simulink model "torqueBalancing2015a"  (Simulink 8.5)
settings: Solver=FixedStepDiscrete  StartTime=0.0  StopTime="CONFIG.SIMULATION_TIME "  FixedStep=CONFIG.Ts  RelTol=1e-3
InitFcn:
  | cd(fileparts(which(bdroot)));
  | initTorqueBalancing;
values from neighbouring files (symbols this model uses):
  WBT_modelName = 'matlabTorqueBalancing'    [initTorqueBalancing.m]
undefined symbols (not defined in the file or in its folder): bVectorConstraintsFeet, bVectorConstraintsLegs, CONFIG, ConstraintsMatrixFeet, ConstraintsMatrixLegs, DiscIntNeverNeededParam, gain, references, reg, ROBOT_DOF, ROBOT_DOF_FOR_SIMULINK, sat, SM, sm, WBT_robotName
libraries: WBToolboxLibrary x177, simulink x13
(part 4 of 4)

== system torqueBalancing2015a/DesValues/State Machine StandUp/visualise inertial/l_sole_H_root_link3 ==
  qj : Inport
  Constant5 : Constant  Value=eye(4)
  Constant6 : Constant  Value=eye(4)
  Inv\* : Product  Inputs=/*  Multiplication=Matrix(*)
  Visualize hom transf4 : Subsystem
  link_name : WBToolboxLibrary/wholeBodyModel/Kinematics/Forward Kinematics  frameName=link_name  robotName=WBT_robotName  localName=WBT_modelName  wbiFile=WBT_wbiFilename  wbiList=WBT_wbiList
  root_link : WBToolboxLibrary/wholeBodyModel/Kinematics/Forward Kinematics  frameName='root_link'  robotName=WBT_robotName  localName=WBT_modelName  wbiFile=WBT_wbiFilename  wbiList=WBT_wbiList
  link_name_H_root_link : Outport
  wires:
  Constant5/1 -> link_name/1
  Inv\*/1 -> link_name_H_root_link/1  "link_name_H_root_link"
  link_name/1 -> Inv\*/1
  Constant6/1 -> root_link/1
  qj/1 -> link_name/2, root_link/2
  root_link/1 -> Visualize hom transf4/1(H), Inv\*/2

== system torqueBalancing2015a/DesValues/State Machine StandUp/visualise inertial/w_H_root_link1 ==
  qj : Inport
  inertial : Inport  Port=2
  "CoM6D ->  CoMXYZ1" : Selector  NumberOfDimensions=2  InputPortWidth=7  IndexOptions=Index vector (dialog),Index vector (dialog)  Indices=[1 2 3],[1 2 3]  OutputSizes=1,1
  Constant : Constant  Value=zeros(3,1)
  Constant2 : Constant  Value=eye(4)
  Constant5 : Constant  Value=eye(4)
  Constant6 : Constant  Value=eye(4)
  Gain : Gain  Gain=pi/180
  Head state : WBToolboxLibrary/Utilities/Yarp Read  portName=[WBT_robotName, '/head/state:o']  signalSize=6  blocking=off  timestamp=off  autoconnect=on  errorOnConnection=off
  Inv\* : Product  Inputs=/*  Multiplication=Matrix(*)
  Inv\*1 : Product  Inputs=/*  Multiplication=Matrix(*)
  Inv\*2 : Product  Inputs=/  Multiplication=Matrix(*)
  Product : Product  Multiplication=Matrix(*)
  Selector : Selector  InputPortWidth=12  IndexOptions=Index vector (dialog)  Indices=[4 5 6 ]  OutputSizes=1
  Selector1 : Selector  InputPortWidth=6  IndexOptions=Index vector (dialog)  Indices=[1:3]  OutputSizes=1
  Switch : Switch  Criteria=u2 > Threshold
  Switch6 : Switch  Criteria=u2 > Threshold
  USE_IMU4EST_BASE : Constant  Value=CONFIG.USE_IMU4EST_BASE
  USE_IMU4EST_BASE1 : Constant  Value=CONFIG.CORRECT_NECK_IMU
  fromImuToHomogeousTransformFCN : MATLAB Function  TreatAsAtomicUnit=on
      settings: PermitHierarchicalResolution=ParametersOnly
  holder 1 : WBToolboxLibrary/Utilities/holder 
  holder 2 : WBToolboxLibrary/Utilities/holder 
  imu : WBToolboxLibrary/wholeBodyModel/Kinematics/Forward Kinematics  frameName='imu_frame'  robotName=WBT_robotName  localName=WBT_modelName  wbiFile=WBT_wbiFilename  wbiList=WBT_wbiList
  l_sole_acc : Scope
      settings: TimeRange=60  ShowLegends=on  MaxDataPoints=5000  SaveToWorkspace=off  YMin=-4.47309  YMax=14.2668  SampleTime=-1
  link : WBToolboxLibrary/wholeBodyModel/Kinematics/Forward Kinematics  frameName=link_name  robotName=WBT_robotName  localName=WBT_modelName  wbiFile=WBT_wbiFilename  wbiList=WBT_wbiList
  root_link : WBToolboxLibrary/wholeBodyModel/Kinematics/Forward Kinematics  frameName='root_link'  robotName=WBT_robotName  localName=WBT_modelName  wbiFile=WBT_wbiFilename  wbiList=WBT_wbiList
  w_H_root : Outport
  wires:
  Constant5/1 -> imu/1
  Inv\*/1 -> Inv\*2/1, holder 1/1, fromImuToHomogeousTransformFCN/1(imu_H_link)  "imu_H_link"
  imu/1 -> Inv\*/1
  Constant6/1 -> link/1
  Inv\*1/1 -> Switch6/3, fromImuToHomogeousTransformFCN/3(link_H_root)  "link_H_root"
  link/1 -> Inv\*/2, Inv\*1/1
  inertial/1 -> Selector/1, holder 2/1, fromImuToHomogeousTransformFCN/5(inertial)
  Switch6/1 -> w_H_root/1
  USE_IMU4EST_BASE/1 -> Switch6/2
  fromImuToHomogeousTransformFCN/1(w_H_root) -> Switch6/1
  Constant2/1 -> root_link/1
  qj/1 -> root_link/2, link/2, imu/2
  root_link/1 -> Inv\*1/2
  holder 1/1 -> fromImuToHomogeousTransformFCN/2(imu_H_link_0)
  holder 2/1 -> fromImuToHomogeousTransformFCN/4(inertial_0)
  Inv\*2/1 -> "CoM6D ->  CoMXYZ1"/1
  "CoM6D ->  CoMXYZ1"/1 -> Product/1  "l_sole_R_imu"
  Selector/1 -> Product/2  "imu_acce"
  Product/1 -> l_sole_acc/1
  Head state/1 -> Gain/1
  Selector1/1 -> Switch/1  "neck"
  USE_IMU4EST_BASE1/1 -> Switch/2
  Switch/1 -> fromImuToHomogeousTransformFCN/6(neck)
  Gain/1 -> Selector1/1
  Constant/1 -> Switch/3

== system torqueBalancing2015a/DesValues/State Machine StandUp/visualise inertial/w_H_root_link4 ==
  qj : Inport
  inertial : Inport  Port=2
  "CoM6D ->  CoMXYZ1" : Selector  NumberOfDimensions=2  InputPortWidth=7  IndexOptions=Index vector (dialog),Index vector (dialog)  Indices=[1 2 3],[1 2 3]  OutputSizes=1,1
  Constant : Constant  Value=zeros(3,1)
  Constant2 : Constant  Value=eye(4)
  Constant5 : Constant  Value=eye(4)
  Constant6 : Constant  Value=eye(4)
  Gain : Gain  Gain=pi/180
  Head state : WBToolboxLibrary/Utilities/Yarp Read  portName=[WBT_robotName, '/head/state:o']  signalSize=6  blocking=off  timestamp=off  autoconnect=on  errorOnConnection=off
  Inv\* : Product  Inputs=/*  Multiplication=Matrix(*)
  Inv\*1 : Product  Inputs=/*  Multiplication=Matrix(*)
  Inv\*2 : Product  Inputs=/  Multiplication=Matrix(*)
  Product : Product  Multiplication=Matrix(*)
  Selector : Selector  InputPortWidth=12  IndexOptions=Index vector (dialog)  Indices=[4 5 6 ]  OutputSizes=1
  Selector1 : Selector  InputPortWidth=6  IndexOptions=Index vector (dialog)  Indices=[1:3]  OutputSizes=1
  Switch : Switch  Criteria=u2 > Threshold
  Switch6 : Switch  Criteria=u2 > Threshold
  USE_IMU4EST_BASE : Constant  Value=CONFIG.USE_IMU4EST_BASE
  USE_IMU4EST_BASE1 : Constant  Value=CONFIG.CORRECT_NECK_IMU
  fromImuToHomogeousTransformFCN : MATLAB Function  TreatAsAtomicUnit=on
      settings: PermitHierarchicalResolution=ParametersOnly
  holder 1 : WBToolboxLibrary/Utilities/holder 
  holder 2 : WBToolboxLibrary/Utilities/holder 
  imu : WBToolboxLibrary/wholeBodyModel/Kinematics/Forward Kinematics  frameName='imu_frame'  robotName=WBT_robotName  localName=WBT_modelName  wbiFile=WBT_wbiFilename  wbiList=WBT_wbiList
  l_sole_acc : Scope
      settings: TimeRange=60  ShowLegends=on  MaxDataPoints=5000  SaveToWorkspace=off  YMin=-4.47309  YMax=14.2668  SampleTime=-1
  link : WBToolboxLibrary/wholeBodyModel/Kinematics/Forward Kinematics  frameName=link_name  robotName=WBT_robotName  localName=WBT_modelName  wbiFile=WBT_wbiFilename  wbiList=WBT_wbiList
  root_link : WBToolboxLibrary/wholeBodyModel/Kinematics/Forward Kinematics  frameName='root_link'  robotName=WBT_robotName  localName=WBT_modelName  wbiFile=WBT_wbiFilename  wbiList=WBT_wbiList
  w_H_root : Outport
  wires:
  Constant5/1 -> imu/1
  Inv\*/1 -> Inv\*2/1, holder 1/1, fromImuToHomogeousTransformFCN/1(imu_H_link)  "imu_H_link"
  imu/1 -> Inv\*/1
  Constant6/1 -> link/1
  Inv\*1/1 -> Switch6/3, fromImuToHomogeousTransformFCN/3(link_H_root)  "link_H_root"
  link/1 -> Inv\*/2, Inv\*1/1
  inertial/1 -> Selector/1, holder 2/1, fromImuToHomogeousTransformFCN/5(inertial)
  Switch6/1 -> w_H_root/1
  USE_IMU4EST_BASE/1 -> Switch6/2
  fromImuToHomogeousTransformFCN/1(w_H_root) -> Switch6/1
  Constant2/1 -> root_link/1
  qj/1 -> root_link/2, link/2, imu/2
  root_link/1 -> Inv\*1/2
  holder 1/1 -> fromImuToHomogeousTransformFCN/2(imu_H_link_0)
  holder 2/1 -> fromImuToHomogeousTransformFCN/4(inertial_0)
  Inv\*2/1 -> "CoM6D ->  CoMXYZ1"/1
  "CoM6D ->  CoMXYZ1"/1 -> Product/1  "l_sole_R_imu"
  Selector/1 -> Product/2  "imu_acce"
  Product/1 -> l_sole_acc/1
  Head state/1 -> Gain/1
  Selector1/1 -> Switch/1  "neck"
  USE_IMU4EST_BASE1/1 -> Switch/2
  Switch/1 -> fromImuToHomogeousTransformFCN/6(neck)
  Gain/1 -> Selector1/1
  Constant/1 -> Switch/3

== system torqueBalancing2015a/DesValues/State Machine/visualise inertial/l_sole_H_root_link2/Visualize hom transf4 ==
  H : Inport
  "CoM6D ->  CoMXYZ1" : Selector  NumberOfDimensions=2  InputPortWidth=7  IndexOptions=Index vector (dialog),Index vector (dialog)  Indices=[1 2 3],[1 2 3]  OutputSizes=1,1
  "CoM6D ->  CoMXYZ2" : Selector  NumberOfDimensions=2  InputPortWidth=7  IndexOptions=Index vector (dialog),Index vector (dialog)  Indices=[1 2 3],[4]  OutputSizes=1,1
  Hom : Scope
      settings: TimeRange=auto  ShowLegends=on  MaxDataPoints=5000  SaveToWorkspace=off  SaveName=ScopeData3  YMin=-1.25  YMax=1.25  SampleTime=-1
  R : Scope
      settings: TimeRange=auto  MaxDataPoints=5000  SaveToWorkspace=off  YMin=-0.125  YMax=1.125  SampleTime=-1
  p : Scope
      settings: TimeRange=auto  MaxDataPoints=5000  SaveToWorkspace=off  SaveName=ScopeData2  YMin=-1.00000  YMax=1.00000  SampleTime=-1
  wires:
  "CoM6D ->  CoMXYZ1"/1 -> R/1
  "CoM6D ->  CoMXYZ2"/1 -> p/1
  H/1 -> "CoM6D ->  CoMXYZ2"/1, Hom/1, "CoM6D ->  CoMXYZ1"/1

== system torqueBalancing2015a/DesValues/State Machine/visualise inertial/l_sole_H_root_link3/Visualize hom transf4 ==
  H : Inport
  "CoM6D ->  CoMXYZ1" : Selector  NumberOfDimensions=2  InputPortWidth=7  IndexOptions=Index vector (dialog),Index vector (dialog)  Indices=[1 2 3],[1 2 3]  OutputSizes=1,1
  "CoM6D ->  CoMXYZ2" : Selector  NumberOfDimensions=2  InputPortWidth=7  IndexOptions=Index vector (dialog),Index vector (dialog)  Indices=[1 2 3],[4]  OutputSizes=1,1
  Hom : Scope
      settings: TimeRange=auto  ShowLegends=on  MaxDataPoints=5000  SaveToWorkspace=off  SaveName=ScopeData3  YMin=-1.25  YMax=1.25  SampleTime=-1
  R : Scope
      settings: TimeRange=auto  MaxDataPoints=5000  SaveToWorkspace=off  YMin=-0.125  YMax=1.125  SampleTime=-1
  p : Scope
      settings: TimeRange=auto  MaxDataPoints=5000  SaveToWorkspace=off  SaveName=ScopeData2  YMin=-1.00000  YMax=1.00000  SampleTime=-1
  wires:
  "CoM6D ->  CoMXYZ1"/1 -> R/1
  "CoM6D ->  CoMXYZ2"/1 -> p/1
  H/1 -> "CoM6D ->  CoMXYZ2"/1, Hom/1, "CoM6D ->  CoMXYZ1"/1

== system torqueBalancing2015a/DesValues/State Machine StandUp/visualise inertial/l_sole_H_root_link2/Visualize hom transf4 ==
  H : Inport
  "CoM6D ->  CoMXYZ1" : Selector  NumberOfDimensions=2  InputPortWidth=7  IndexOptions=Index vector (dialog),Index vector (dialog)  Indices=[1 2 3],[1 2 3]  OutputSizes=1,1
  "CoM6D ->  CoMXYZ2" : Selector  NumberOfDimensions=2  InputPortWidth=7  IndexOptions=Index vector (dialog),Index vector (dialog)  Indices=[1 2 3],[4]  OutputSizes=1,1
  Hom : Scope
      settings: TimeRange=auto  ShowLegends=on  MaxDataPoints=5000  SaveToWorkspace=off  SaveName=ScopeData3  YMin=-1.25  YMax=1.25  SampleTime=-1
  R : Scope
      settings: TimeRange=auto  MaxDataPoints=5000  SaveToWorkspace=off  YMin=-0.125  YMax=1.125  SampleTime=-1
  p : Scope
      settings: TimeRange=auto  MaxDataPoints=5000  SaveToWorkspace=off  SaveName=ScopeData2  YMin=-1.00000  YMax=1.00000  SampleTime=-1
  wires:
  "CoM6D ->  CoMXYZ1"/1 -> R/1
  "CoM6D ->  CoMXYZ2"/1 -> p/1
  H/1 -> "CoM6D ->  CoMXYZ2"/1, Hom/1, "CoM6D ->  CoMXYZ1"/1

== system torqueBalancing2015a/DesValues/State Machine StandUp/visualise inertial/l_sole_H_root_link3/Visualize hom transf4 ==
  H : Inport
  "CoM6D ->  CoMXYZ1" : Selector  NumberOfDimensions=2  InputPortWidth=7  IndexOptions=Index vector (dialog),Index vector (dialog)  Indices=[1 2 3],[1 2 3]  OutputSizes=1,1
  "CoM6D ->  CoMXYZ2" : Selector  NumberOfDimensions=2  InputPortWidth=7  IndexOptions=Index vector (dialog),Index vector (dialog)  Indices=[1 2 3],[4]  OutputSizes=1,1
  Hom : Scope
      settings: TimeRange=auto  ShowLegends=on  MaxDataPoints=5000  SaveToWorkspace=off  SaveName=ScopeData3  YMin=-1.25  YMax=1.25  SampleTime=-1
  R : Scope
      settings: TimeRange=auto  MaxDataPoints=5000  SaveToWorkspace=off  YMin=-0.125  YMax=1.125  SampleTime=-1
  p : Scope
      settings: TimeRange=auto  MaxDataPoints=5000  SaveToWorkspace=off  SaveName=ScopeData2  YMin=-1.00000  YMax=1.00000  SampleTime=-1
  wires:
  "CoM6D ->  CoMXYZ1"/1 -> R/1
  "CoM6D ->  CoMXYZ2"/1 -> p/1
  H/1 -> "CoM6D ->  CoMXYZ2"/1, Hom/1, "CoM6D ->  CoMXYZ1"/1

== matlab function DesValues/State Machine/visualise inertial/w_H_root_link1/fromImuToHomogeousTransformFCN ==
  data: imu_H_link input double; imu_H_link_0 input double; link_H_root input double; inertial_0 input double; inertial input double; neck input double; w_H_root output double; CONFIG parameter double
function w_H_root = fromBaseToWorldWithImuFCN(imu_H_link,imu_H_link_0,link_H_root,inertial_0,inertial,neck,CONFIG)
%#codegen
w_H_root = fromBaseToWorldWithImu(imu_H_link,imu_H_link_0,link_H_root,inertial_0,inertial,neck,CONFIG);

== matlab function DesValues/Internal coordinator/w_H_root_link4/fromImuToHomogeousTransformFCN ==
  data: imu_H_link input double; imu_H_link_0 input double; link_H_root input double; inertial_0 input double; inertial input double; neck input double; w_H_root output double; CONFIG parameter double
function w_H_root = fromBaseToWorldWithImuFCN(imu_H_link,imu_H_link_0,link_H_root,inertial_0,inertial,neck,CONFIG)
%#codegen
w_H_root = fromBaseToWorldWithImu(imu_H_link,imu_H_link_0,link_H_root,inertial_0,inertial,neck,CONFIG);

== matlab function DesValues/State Machine StandUp/Visualise extrnal wrenches  /MATLAB Function ==
  data: state input double; thresholdContactLeft output double; thresholdContactRight output double; sm parameter double
function [thresholdContactLeft,thresholdContactRight] = fcn(state,sm)

    thresholdContactLeft  = sm.LwrenchThreshold(state);
    thresholdContactRight = sm.RwrenchThreshold(state);

end

== matlab function controller_QP/integralOf Hw1/MATLAB Function ==
  data: qjErr input double; JL input double; JR input double; vbEquivalent output double; reg parameter double; activeFeetConstraints input double
 function vbEquivalent = generateReferencesForH(qjErr,JL,JR,reg,activeFeetConstraints)
%#codegen
if activeFeetConstraints(1) == 1
    
    pinvJb             = (JL(:,1:6)'*JL(:,1:6) + reg.pinvDampVb*eye(6))\JL(:,1:6)';
    vbEquivalent       = -pinvJb*JL(:,7:end)*qjErr;
else
    
    pinvJb             = (JR(:,1:6)'*JR(:,1:6) + reg.pinvDampVb*eye(6))\JR(:,1:6)';
    vbEquivalent       = -pinvJb*JR(:,7:end)*qjErr;
end
    
end

== matlab function DesValues/State Machine Walking/nu/MATLAB Function ==
  data: JcLeftFoot input double; JcRightFoot input double; activeFeetConstraints input double; y output double; qD input double; reg parameter double
function y = fcn(JcLeftFoot,JcRightFoot,activeFeetConstraints,qD,reg)
%#codegen

Jc = [activeFeetConstraints(1)*JcLeftFoot;
      activeFeetConstraints(2)*JcRightFoot];

pinvJb = (Jc(:,1:6)'*Jc(:,1:6) + reg.pinvDampVb*eye(6))\Jc(:,1:6)';  
  
% pinvJb = pinv(Jc(:,1:6));

y = -pinvJb*Jc(:,7:end)*qD;

== matlab function DesValues/State Machine Walking/stateMachineFCN ==
  data: connection input double; wrench_rightFoot input double; wrench_leftFoot input double; CoM_0 input double; q0 input double; w_CoM input double; CoMIn input double; qIn input double; constraintsIn input double; w_H_b output double; CoMDes output double; qDes output double; constraints output double; l_sole_H_b input double; r_sole_H_b input double; sm parameter double; impedances output double; gain parameter double; currentState output double
function [w_H_b, CoMDes,qDes,constraints,impedances,currentState] = ...
    stateMachineFCN(connection,wrench_rightFoot,wrench_leftFoot,CoM_0, q0, w_CoM , CoMIn, qIn, constraintsIn, l_sole_H_b, r_sole_H_b, sm,gain)
%#codegen
 
[CoMDes,qDes,constraints, currentState,impedances,w_H_b] = ...
    stateMachineWalking(connection,CoM_0, q0, w_CoM, CoMIn, qIn, constraintsIn, wrench_rightFoot,wrench_leftFoot,l_sole_H_b, r_sole_H_b, sm,gain);

== matlab function DesValues/Internal coordinator/nu/MATLAB Function ==
  data: JcLeftFoot input double; JcRightFoot input double; activeFeetConstraints input double; y output double; qD input double; reg parameter double
function y = fcn(JcLeftFoot,JcRightFoot,activeFeetConstraints,qD,reg)
%#codegen

Jc = [activeFeetConstraints(1)*JcLeftFoot;
      activeFeetConstraints(2)*JcRightFoot];

pinvJb = (Jc(:,1:6)'*Jc(:,1:6) + reg.pinvDampVb*eye(6))\Jc(:,1:6)';  
  
% pinvJb = pinv(Jc(:,1:6));

y = -pinvJb*Jc(:,7:end)*qD;

== matlab function DesValues/State Machine/w_H_root_link4/fromImuToHomogeousTransformFCN ==
  data: imu_H_link input double; imu_H_link_0 input double; link_H_root input double; inertial_0 input double; inertial input double; neck input double; w_H_root output double; CONFIG parameter double
function w_H_root = fromBaseToWorldWithImuFCN(imu_H_link,imu_H_link_0,link_H_root,inertial_0,inertial,neck,CONFIG)
%#codegen
w_H_root = fromBaseToWorldWithImu(imu_H_link,imu_H_link_0,link_H_root,inertial_0,inertial,neck,CONFIG);

== matlab function DesValues/State Machine/w_H_root_link1/fromImuToHomogeousTransformFCN ==
  data: imu_H_link input double; imu_H_link_0 input double; link_H_root input double; inertial_0 input double; inertial input double; neck input double; w_H_root output double; CONFIG parameter double
function w_H_root = fromBaseToWorldWithImuFCN(imu_H_link,imu_H_link_0,link_H_root,inertial_0,inertial,neck,CONFIG)
%#codegen
w_H_root = fromBaseToWorldWithImu(imu_H_link,imu_H_link_0,link_H_root,inertial_0,inertial,neck,CONFIG);

== matlab function DesValues/Internal coordinator/refGen/refGenFCN ==
  data: xCom0 input double; qDes output double; q0 input double; t input double; references parameter double; desired_x_dx_ddx_CoM output double
function [qDes,desired_x_dx_ddx_CoM] = refGenFCN(xCom0,q0,t,references)
%#codegen

[qDes,desired_x_dx_ddx_CoM] = refGen(xCom0,q0,t,references);

== matlab function DesValues/State Machine Walking/w_H_root_link4/fromImuToHomogeousTransformFCN ==
  data: imu_H_link input double; imu_H_link_0 input double; link_H_root input double; inertial_0 input double; inertial input double; neck input double; w_H_root output double; CONFIG parameter double
function w_H_root = fromBaseToWorldWithImuFCN(imu_H_link,imu_H_link_0,link_H_root,inertial_0,inertial,neck,CONFIG)
%#codegen
w_H_root = fromBaseToWorldWithImu(imu_H_link,imu_H_link_0,link_H_root,inertial_0,inertial,neck,CONFIG);

== matlab function DesValues/State Machine/nu/MATLAB Function ==
  data: JcLeftFoot input double; JcRightFoot input double; activeFeetConstraints input double; y output double; qD input double; reg parameter double
function y = fcn(JcLeftFoot,JcRightFoot,activeFeetConstraints,qD,reg)
%#codegen

Jc = [activeFeetConstraints(1)*JcLeftFoot;
      activeFeetConstraints(2)*JcRightFoot];

pinvJb = pinvDamped(Jc(:,1:6),reg.pinvDampVb);  
  
% pinvJb = pinv(Jc(:,1:6));

y = -pinvJb*Jc(:,7:end)*qD;

== matlab function DesValues/State Machine/stateMachineFCN ==
  data: wrench_rightFoot input double; wrench_leftFoot input double; w_H_b output double; CoMDes output double; qDes output double; constraints output double; CoM_0 input double; q0 input double; l_sole_CoM input double; r_sole_CoM input double; qj input double; t input double; l_sole_H_b input double; r_sole_H_b input double; sm parameter double; impedances output double; kpCom output double; kdCom output double; gain parameter double; currentState output double; jointsSmoothingTime output double
function [w_H_b, CoMDes,qDes,constraints,impedances,kpCom,kdCom,currentState,jointsSmoothingTime] = ...
    stateMachineFCN(wrench_rightFoot,wrench_leftFoot,CoM_0, q0, l_sole_CoM,r_sole_CoM,qj, t, l_sole_H_b, r_sole_H_b, sm,gain)

%#codegen
[w_H_b, CoMDes,qDes,constraints,impedances,kpCom,kdCom,currentState,jointsSmoothingTime] = ...
    stateMachine(CoM_0,q0,l_sole_CoM,r_sole_CoM,qj,t,wrench_rightFoot,wrench_leftFoot,l_sole_H_b,r_sole_H_b, sm,gain); 

end

== matlab function DesValues/State Machine Walking/w_H_root_link1/fromImuToHomogeousTransformFCN ==
  data: imu_H_link input double; imu_H_link_0 input double; link_H_root input double; inertial_0 input double; inertial input double; neck input double; w_H_root output double; CONFIG parameter double
function w_H_root = fromBaseToWorldWithImuFCN(imu_H_link,imu_H_link_0,link_H_root,inertial_0,inertial,neck,CONFIG)
%#codegen
w_H_root = fromBaseToWorldWithImu(imu_H_link,imu_H_link_0,link_H_root,inertial_0,inertial,neck,CONFIG);

== matlab function Dump and visualize/plotNorms/norm ==
  data: u input double; normU output double
function normU = fcn(u)
%#codegen

normU = norm(u);

== matlab function Dump and visualize/plotNorms/norm1 ==
  data: u input double; normU output double
function normU = fcn(u)
%#codegen

normU = norm(u);

== matlab function controller_QP/tau(f)  ==
  data: tauModel output double; Sigma output double; NA output double; fHdotDesC1C2 output double; HessianMatrixQP1Foot output double; gradientQP1Foot output double; ConstraintsMatrixQP1Foot output double; bVectorConstraintsQp1Foot output double; HessianMatrixQP2FeetOrLegs output double; gradientQP2FeetOrLegs output double; ConstraintsMatrixQP2FeetOrLegs output double; bVectorConstraintsQp2FeetOrLegs output double; constraints input double; ROBOT_DOF_FOR_SIMULINK input double; ConstraintsMatrix input double; bVectorConstraints input double; q input double; qDes input double; v input double; M input double; h input double; H input double; intHw input double; w_H_l_contact input double; w_H_r_contact input double; JL input double; JR input double; dJLv input double; dJRv input double; xcom input double; J_CoM input double; desired_x_dx_ddx_CoM input double; gainsPCOM input double; gainsDCOM input double; impedances input double; intErrorCoM input double; ki_int_qtilde input double; reg parameter double; gain parameter double; errorCoM output double; qTilde output double; f output double; w_H_lArm input double; w_H_rArm input double; LArmWrench input double; RArmWrench input double; useExtArmForces input double; correctionFromSupportForce output double; H_error output double; V output double
function [tauModel,Sigma,NA,fHdotDesC1C2, ...
          HessianMatrixQP1Foot,gradientQP1Foot,ConstraintsMatrixQP1Foot,bVectorConstraintsQp1Foot,...
          HessianMatrixQP2FeetOrLegs,gradientQP2FeetOrLegs,ConstraintsMatrixQP2FeetOrLegs,bVectorConstraintsQp2FeetOrLegs,...
          errorCoM,qTilde,f,correctionFromSupportForce,H_error,V]    =  ...
          balancingControllerFCN(constraints,ROBOT_DOF_FOR_SIMULINK,ConstraintsMatrix,bVectorConstraints,...
          q,qDes,v,M,h,H,intHw,w_H_l_contact,w_H_r_contact,JL,JR,dJLv,dJRv,xcom,J_CoM,desired_x_dx_ddx_CoM,...
          gainsPCOM,gainsDCOM,impedances,intErrorCoM,ki_int_qtilde,reg,gain,...
          w_H_lArm,w_H_rArm,LArmWrench,RArmWrench,useExtArmForces)
      
%#codegen

          [tauModel,Sigma,NA,fHdotDesC1C2, ...
           HessianMatrixQP1Foot,gradientQP1Foot,ConstraintsMatrixQP1Foot,bVectorConstraintsQp1Foot,...
           HessianMatrixQP2FeetOrLegs,gradientQP2FeetOrLegs,ConstraintsMatrixQP2FeetOrLegs,bVectorConstraintsQp2FeetOrLegs,...
           errorCoM,qTilde,f,correctionFromSupportForce,H_error,V]    =  ...
           balancingController(constraints,ROBOT_DOF_FOR_SIMULINK,ConstraintsMatrix,bVectorConstraints,...
           q,qDes,v,M,h,H,intHw,w_H_l_contact,w_H_r_contact,JL,JR, dJLv,dJRv,xcom,J_CoM,desired_x_dx_ddx_CoM,...
           gainsPCOM,gainsDCOM,impedances,intErrorCoM,ki_int_qtilde,reg,gain,...
           w_H_lArm,w_H_rArm,LArmWrench,RArmWrench,useExtArmForces);
end

== matlab function emergency stop: joint limits/MATLAB Function ==
  data: umin input double; umax input double; u input double; inRange output double; tol input double
function inRange = checkRange(umin, umax, u, tol)
%#codegen

res = u < umin + tol | u > umax - tol;
res = sum(res);
if res==0
    inRange = 1;
else
    inRange = 0;
    u < umin + tol | u > umax - tol
end

== matlab function DesValues/State Machine StandUp/nu/MATLAB Function ==
  data: JcLeftFoot input double; JcRightFoot input double; activeFeetConstraints input double; y output double; qD input double; reg parameter double
function y = fcn(JcLeftFoot,JcRightFoot,activeFeetConstraints,qD,reg)
%#codegen

Jc = [activeFeetConstraints(1)*JcLeftFoot;
      activeFeetConstraints(2)*JcRightFoot];

pinvJb = pinvDamped(Jc(:,1:6),reg.pinvDampVb);  
  
% pinvJb = pinv(Jc(:,1:6));

y = -pinvJb*Jc(:,7:end)*qD;

== matlab function DesValues/State Machine StandUp/stateMachineFCN ==
  data: qjRef input double; CoM input double; CoM_0 input double; l_sole_H_b input double; l_upper_leg_contact_H_b input double; w_H_b output double; constraints output double; t input double; impedances output double; kpCom output double; kdCom output double; gain parameter double; currentState output double; jointsSmoothingTime output double; sm parameter double; qjDes output double; CoM_Des output double; Lwrench input double; Rwrench input double; LHandWrench input double; RHandWrench input double; useExtArmForces input double
function  [w_H_b,constraints,impedances,kpCom,kdCom,currentState,jointsSmoothingTime,qjDes,CoM_Des] = ...
          stateMachineStandUpFCN(qjRef,CoM,CoM_0,l_sole_H_b,l_upper_leg_contact_H_b,t,gain,sm,Lwrench,Rwrench,LHandWrench,RHandWrench,useExtArmForces)
%#codegen
 [w_H_b,constraints,impedances,kpCom,kdCom,currentState,jointsSmoothingTime,qjDes,CoM_Des] = ...
  stateMachineStandUp(qjRef,CoM,CoM_0,l_sole_H_b,l_upper_leg_contact_H_b,t,gain,sm,Lwrench,Rwrench,LHandWrench,RHandWrench,useExtArmForces);

end

== matlab function controller_QP/MATLAB Function ==
  data: icubStandup input double; legsInContact output double; state input double
function legsInContact = contactDetectorFCN(icubStandup,state)

legsInContact = contactDetector(icubStandup,state);

end

== matlab function DesValues/State Machine/visualise inertial/Visualize hom transf2/MATLAB Function ==
  data: R input double; rollPitchYaw output double
function rollPitchYaw = buildHomogenousTranformation(R)
%#codegen

rollPitchYaw = rollPitchYawFromRotation(R);

rollPitchYaw = rollPitchYaw*180/pi;

== matlab function DesValues/State Machine/visualise inertial/Visualize hom transf4/MATLAB Function ==
  data: R input double; rollPitchYaw output double
function rollPitchYaw = buildHomogenousTranformation(R)
%#codegen

rollPitchYaw = rollPitchYawFromRotation(R);

rollPitchYaw = rollPitchYaw*180/pi;

== matlab function DesValues/State Machine/visualise inertial/Visualize hom transf5/MATLAB Function ==
  data: R input double; rollPitchYaw output double
function rollPitchYaw = buildHomogenousTranformation(R)
%#codegen

rollPitchYaw = rollPitchYawFromRotation(R);

rollPitchYaw = rollPitchYaw*180/pi;

== matlab function DesValues/State Machine/visualise inertial/Visualize hom transf6/MATLAB Function ==
  data: R input double; rollPitchYaw output double
function rollPitchYaw = buildHomogenousTranformation(R)
%#codegen

rollPitchYaw = rollPitchYawFromRotation(R);

rollPitchYaw = rollPitchYaw*180/pi;

== matlab function controller_QP/integralOf Hw1/w_H_root_link4/fromImuToHomogeousTransformFCN ==
  data: imu_H_link input double; imu_H_link_0 input double; link_H_root input double; inertial_0 input double; inertial input double; neck input double; w_H_root output double; CONFIG parameter double
function w_H_root = fromBaseToWorldWithImuFCN(imu_H_link,imu_H_link_0,link_H_root,inertial_0,inertial,neck,CONFIG)
%#codegen
w_H_root = fromBaseToWorldWithImu(imu_H_link,imu_H_link_0,link_H_root,inertial_0,inertial,neck,CONFIG);

== matlab function DesValues/State Machine/visualise inertial/w_H_root_link4/fromImuToHomogeousTransformFCN ==
  data: imu_H_link input double; imu_H_link_0 input double; link_H_root input double; inertial_0 input double; inertial input double; neck input double; w_H_root output double; CONFIG parameter double
function w_H_root = fromBaseToWorldWithImuFCN(imu_H_link,imu_H_link_0,link_H_root,inertial_0,inertial,neck,CONFIG)
%#codegen
w_H_root = fromBaseToWorldWithImu(imu_H_link,imu_H_link_0,link_H_root,inertial_0,inertial,neck,CONFIG);

== matlab function DesValues/State Machine StandUp/visualise inertial/Visualize hom transf2/MATLAB Function ==
  data: R input double; rollPitchYaw output double
function rollPitchYaw = buildHomogenousTranformation(R)
%#codegen

rollPitchYaw = rollPitchYawFromRotation(R);

rollPitchYaw = rollPitchYaw*180/pi;

== matlab function DesValues/State Machine StandUp/visualise inertial/Visualize hom transf4/MATLAB Function ==
  data: R input double; rollPitchYaw output double
function rollPitchYaw = buildHomogenousTranformation(R)
%#codegen

rollPitchYaw = rollPitchYawFromRotation(R);

rollPitchYaw = rollPitchYaw*180/pi;

== matlab function DesValues/State Machine StandUp/visualise inertial/Visualize hom transf5/MATLAB Function ==
  data: R input double; rollPitchYaw output double
function rollPitchYaw = buildHomogenousTranformation(R)
%#codegen

rollPitchYaw = rollPitchYawFromRotation(R);

rollPitchYaw = rollPitchYaw*180/pi;

== matlab function DesValues/State Machine StandUp/visualise inertial/Visualize hom transf6/MATLAB Function ==
  data: R input double; rollPitchYaw output double
function rollPitchYaw = buildHomogenousTranformation(R)
%#codegen

rollPitchYaw = rollPitchYawFromRotation(R);

rollPitchYaw = rollPitchYaw*180/pi;

== matlab function DesValues/State Machine StandUp/visualise inertial/Visualize hom transf7/MATLAB Function ==
  data: R input double; rollPitchYaw output double
function rollPitchYaw = buildHomogenousTranformation(R)
%#codegen

rollPitchYaw = rollPitchYawFromRotation(R);

rollPitchYaw = rollPitchYaw*180/pi;

== matlab function DesValues/State Machine StandUp/visualise inertial/Visualize hom transf8/MATLAB Function ==
  data: R input double; rollPitchYaw output double
function rollPitchYaw = buildHomogenousTranformation(R)
%#codegen

rollPitchYaw = rollPitchYawFromRotation(R);

rollPitchYaw = rollPitchYaw*180/pi;

== matlab function DesValues/State Machine StandUp/visualise inertial/w_H_root_link1/fromImuToHomogeousTransformFCN ==
  data: imu_H_link input double; imu_H_link_0 input double; link_H_root input double; inertial_0 input double; inertial input double; neck input double; w_H_root output double; CONFIG parameter double
function w_H_root = fromBaseToWorldWithImuFCN(imu_H_link,imu_H_link_0,link_H_root,inertial_0,inertial,neck,CONFIG)
%#codegen
w_H_root = fromBaseToWorldWithImu(imu_H_link,imu_H_link_0,link_H_root,inertial_0,inertial,neck,CONFIG);

== matlab function DesValues/State Machine StandUp/visualise inertial/w_H_root_link4/fromImuToHomogeousTransformFCN ==
  data: imu_H_link input double; imu_H_link_0 input double; link_H_root input double; inertial_0 input double; inertial input double; neck input double; w_H_root output double; CONFIG parameter double
function w_H_root = fromBaseToWorldWithImuFCN(imu_H_link,imu_H_link_0,link_H_root,inertial_0,inertial,neck,CONFIG)
%#codegen
w_H_root = fromBaseToWorldWithImu(imu_H_link,imu_H_link_0,link_H_root,inertial_0,inertial,neck,CONFIG);

== matlab function DesValues/State Machine StandUp/w_H_root_link1/fromImuToHomogeousTransformFCN ==
  data: imu_H_link input double; imu_H_link_0 input double; link_H_root input double; inertial_0 input double; inertial input double; neck input double; w_H_root output double; CONFIG parameter double
function w_H_root = fromBaseToWorldWithImuFCN(imu_H_link,imu_H_link_0,link_H_root,inertial_0,inertial,neck,CONFIG)
%#codegen
w_H_root = fromBaseToWorldWithImu(imu_H_link,imu_H_link_0,link_H_root,inertial_0,inertial,neck,CONFIG);

== matlab function DesValues/State Machine StandUp/Visualise extrnal wrenches  /MATLAB Function1 ==
  data: state input double; thresholdArmContactLeft output double; thresholdArmContactRight output double; sm parameter double
function [thresholdArmContactLeft,thresholdArmContactRight] = fcn(state,sm)

    thresholdArmContactLeft  = sm.LArmThreshold(state);
    thresholdArmContactRight = sm.RArmThreshold(state);

end

== matlab function DesValues/State Machine/visualise inertial/Visualize hom transf7/MATLAB Function ==
  data: R input double; rollPitchYaw output double
function rollPitchYaw = buildHomogenousTranformation(R)
%#codegen

rollPitchYaw = rollPitchYawFromRotation(R);

rollPitchYaw = rollPitchYaw*180/pi;

== matlab function DesValues/State Machine/visualise inertial/Visualize hom transf8/MATLAB Function ==
  data: R input double; rollPitchYaw output double
function rollPitchYaw = buildHomogenousTranformation(R)
%#codegen

rollPitchYaw = rollPitchYawFromRotation(R);

rollPitchYaw = rollPitchYaw*180/pi;

== matlab function controller_QP/integralOf Hw1/w_H_root_link1/fromImuToHomogeousTransformFCN ==
  data: imu_H_link input double; imu_H_link_0 input double; link_H_root input double; inertial_0 input double; inertial input double; neck input double; w_H_root output double; CONFIG parameter double
function w_H_root = fromBaseToWorldWithImuFCN(imu_H_link,imu_H_link_0,link_H_root,inertial_0,inertial,neck,CONFIG)
%#codegen
w_H_root = fromBaseToWorldWithImu(imu_H_link,imu_H_link_0,link_H_root,inertial_0,inertial,neck,CONFIG);

== matlab function DesValues/State Machine StandUp/w_H_root_link3/fromImuToHomogeousTransformFCN ==
  data: imu_H_link input double; imu_H_link_0 input double; link_H_root input double; inertial_0 input double; inertial input double; neck input double; w_H_root output double; CONFIG parameter double
function w_H_root = fromBaseToWorldWithImuFCN(imu_H_link,imu_H_link_0,link_H_root,inertial_0,inertial,neck,CONFIG)
%#codegen
w_H_root = fromBaseToWorldWithImu(imu_H_link,imu_H_link_0,link_H_root,inertial_0,inertial,neck,CONFIG);
